simulink model "red4_16b"  (R2017a)
settings: Solver=VariableStepAuto  StartTime=0.0  StopTime=10.0  RelTol=1e-3
values from neighbouring files (symbols this model uses):
  alpha = 1    [red_parameters.m]
  beta = 0.7    [red_parameters.m]
  C_river = .017    (= 0.017)    [red_parameters.m]
  C_sea = 0.510    (= 0.51)    [red_parameters.m]
  F = 96485    [red_parameters.m]
  h_river = 60e-6    (= 6e-05)    [red_parameters.m]
  h_sea = 60e-6    (= 6e-05)    [red_parameters.m]
  k_river = 50e-3    (= 0.05)    [red_parameters.m]
  k_sea = 5    [red_parameters.m]
  L = 0.1    [red_parameters.m]
  m_v = 0.0008891    [red_parameters.m]
  Nm = 2    [red_parameters.m]
  R = 8.31    [red_parameters.m]
  R_AEM = R_cl    [red_parameters.m]
  R_CEM = R_Na    [red_parameters.m]
  R_electrodes = 2    [red_parameters.m]
  r_river = 1    [red_parameters.m]
  r_sea = 1    [red_parameters.m]
  SspVsp = 8/h_sea    (= 133333.333333)    [red_parameters.m]
  T = 298    [red_parameters.m]
  t_res = 100    [red_parameters.m]
  z = 1    [red_parameters.m]
undefined symbols (not defined in the file or in its folder): magnitude
libraries: fl_lib x6, nesl_utility x5
settings Model: Creator=root  LastModifiedBy=root

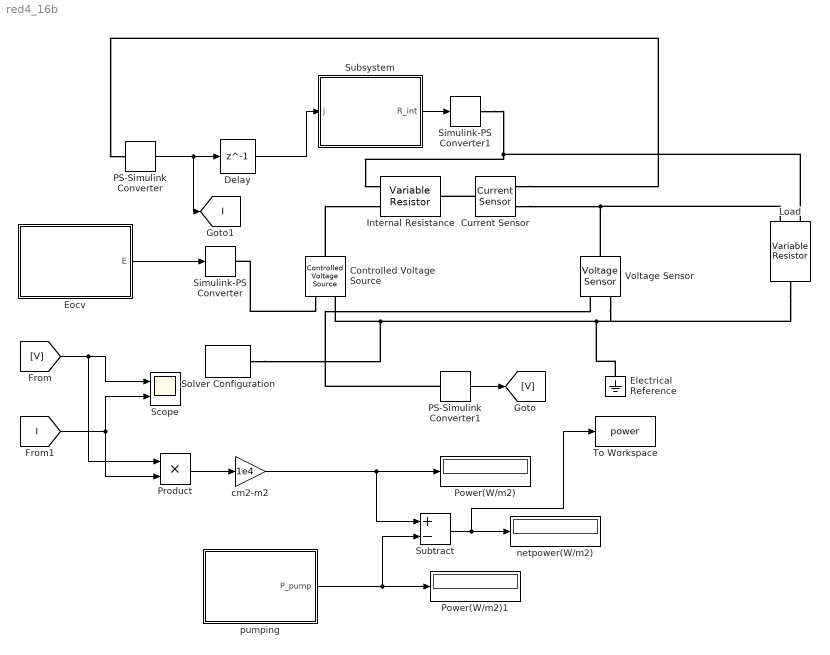
== system red4_16b ==
  Controlled Voltage Source : fl_lib/Electrical/Electrical Sources/Controlled Voltage Source
  Current Sensor : fl_lib/Electrical/Electrical Sensors/Current Sensor
  Delay : Delay  DelayLength=1  InitialCondition=0
  Electrical Reference : fl_lib/Electrical/Electrical Elements/Electrical Reference
  Eocv : Subsystem
  Internal Resistance : fl_lib/Electrical/Electrical Elements/Variable Resistor  Rmin=0 Ohm  i_specify=off  i_priority=None  i=0 A  i_nominal_specify=off  i_nominal_unit=A  i_nominal_value=1  v_specify=off  v_priority=None  v=0 V  v_nominal_specify=off  v_nominal_unit=V  v_nominal_value=1
  Load : fl_lib/Electrical/Electrical Elements/Variable Resistor  Rmin=0 Ohm  i_specify=off  i_priority=None  i=0 A  i_nominal_specify=off  i_nominal_unit=A  i_nominal_value=1  v_specify=off  v_priority=None  v=0 V  v_nominal_specify=off  v_nominal_unit=V  v_nominal_value=1
  PS-Simulink Converter : nesl_utility/PS-Simulink Converter  PhysicalDomain=network_engine_domain  SubClassName=ps_output  LeftPortType=input  RightPortType=output  PseudoPeriodic=off  Frequencies=[]  Unit=1  AffineConversion=off
  PS-Simulink Converter1 : nesl_utility/PS-Simulink Converter  PhysicalDomain=network_engine_domain  SubClassName=ps_output  LeftPortType=input  RightPortType=output  PseudoPeriodic=off  Frequencies=[]  Unit=1  AffineConversion=off
  Power(W/m2) : Display
  Power(W/m2)1 : Display
  Product : Product
  Scope : Scope  NumInputPorts=2
  Simulink-PS Converter : nesl_utility/Simulink-PS Converter  PhysicalDomain=network_engine_domain  SubClassName=ps_input  LeftPortType=input  RightPortType=output  PseudoPeriodic=off  Frequencies=[]  NoiseDistribution=none  NoiseParameters=[]  Unit=1  AffineConversion=off  FilteringAndDerivatives=provide  SimscapeFilterOrder=1  InputFilterTimeConstant=0.001  UdotUserProvided=0
  Simulink-PS Converter1 : nesl_utility/Simulink-PS Converter  PhysicalDomain=network_engine_domain  SubClassName=ps_input  LeftPortType=input  RightPortType=output  PseudoPeriodic=off  Frequencies=[]  NoiseDistribution=none  NoiseParameters=[]  Unit=1  AffineConversion=off  FilteringAndDerivatives=provide  SimscapeFilterOrder=1  InputFilterTimeConstant=0.001  UdotUserProvided=0
  Solver Configuration : nesl_utility/Solver Configuration  PhysicalDomain=network_engine_domain  SubClassName=solver  LeftPortType=input  RightPortType=generic  Accelerate=off  Tones=[]  Harmonics=[]  SimulateNoise=off  Profile=off  UseLocalSampling=off  EnableSwitchedLinearOptims=on  FrequencyDomain=off  UseCCode=off  RelTol=0.001  AbsTol=1e-06  MinStep=1e-09  ToWorkspace=off  RevertToSquareIcSolve=off  NumHomotopyIterations=100  PhasorMode=off  PhasorModeNumHarmonics=1  OverrideAbsTol=off  DoDC=off  ResidualTolerance=1e-09  UseLocalSolver=off  LocalSolverChoice=NE_BACKWARD_EULER_ADVANCER  LocalSolverSampleTime=0.001  DoFixedCost=off  MaxNonlinIter=3  MaxModeIter=2  LinearAlgebra=Sparse  DelaysMemoryBudget=1024  AutomaticFiltering=on  FilteringTimeConstant=0.001
  Subsystem : Subsystem
  Subtract : Sum  Inputs=+-
  To Workspace : ToWorkspace  VariableName=power  SampleTime=1
      settings: MaxDataPoints=1
  Voltage Sensor : fl_lib/Electrical/Electrical Sensors/Voltage Sensor
  cm2-m2 : Gain  Gain=1e4
  netpower(W/m2) : Display
  "pumping " : Subsystem
  tag scope: I=global
  wires:
  Eocv/1(E) -> Simulink-PS Converter/1
  Subsystem/1(R_int) -> Simulink-PS Converter1/1
  PS-Simulink Converter/1 -> [I], Delay/1
  Delay/1 -> Subsystem/1(j)
  PS-Simulink Converter1/1 -> [V]
  [V] -> Product/1, Scope/1
  [I] -> Product/2, Scope/2
  Product/1 -> cm2-m2/1
  cm2-m2/1 -> Subtract/1, Power(W/m2)/1
  "pumping "/1(P_pump) -> Subtract/2, Power(W/m2)1/1
  Subtract/1 -> To Workspace/1, netpower(W/m2)/1
  connections:
  Controlled Voltage Source/RConn1 -- Simulink-PS Converter/RConn1
  Simulink-PS Converter1/RConn1 -- Load/LConn1 -- Internal Resistance/LConn1
  Controlled Voltage Source/LConn1 -- Internal Resistance/LConn2
  Load/RConn1 -- Voltage Sensor/RConn2 -- Electrical Reference/LConn1 -- Solver Configuration/RConn1 -- Controlled Voltage Source/RConn2
  Current Sensor/LConn1 -- Internal Resistance/RConn1
  Current Sensor/RConn2 -- Load/LConn2 -- Voltage Sensor/LConn1
  Current Sensor/RConn1 -- PS-Simulink Converter/LConn1
  PS-Simulink Converter1/LConn1 -- Voltage Sensor/RConn1

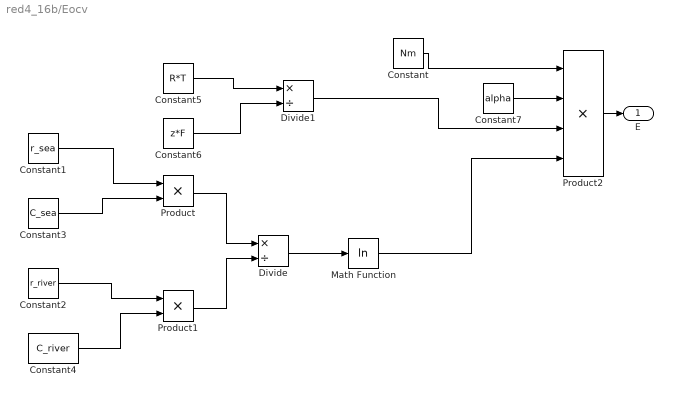
== system red4_16b/Eocv ==
  Constant : Constant  Value=Nm
  Constant1 : Constant  Value=r_sea
  Constant2 : Constant  Value=r_river
  Constant3 : Constant  Value=C_sea
  Constant4 : Constant  Value=C_river
  Constant5 : Constant  Value=R*T
  Constant6 : Constant  Value=z*F
  Constant7 : Constant  Value=alpha
  Divide : Product  Inputs=*/
  Divide1 : Product  Inputs=*/
  Math Function : Math  Operator=log  SaturateOnIntegerOverflow=on
  Product : Product
  Product1 : Product
  Product2 : Product  Inputs=4
  E : Outport
  wires:
  Constant5/1 -> Divide1/1
  Constant1/1 -> Product/1
  Constant4/1 -> Product1/2
  Constant3/1 -> Product/2
  Constant2/1 -> Product1/1
  Product/1 -> Divide/1
  Divide/1 -> Math Function/1
  Product1/1 -> Divide/2
  Constant6/1 -> Divide1/2
  Divide1/1 -> Product2/3
  Math Function/1 -> Product2/4
  Product2/1 -> E/1
  Constant/1 -> Product2/1
  Constant7/1 -> Product2/2

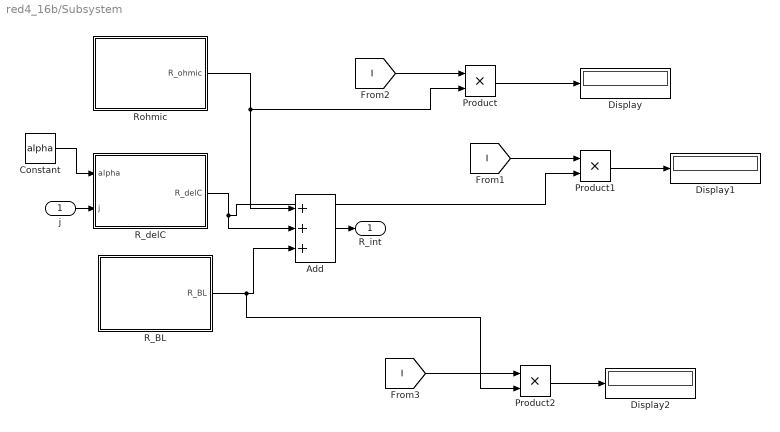
== system red4_16b/Subsystem ==
  j : Inport
  Add : Sum  Inputs=3
  Constant : Constant  Value=alpha
  Display : Display
  Display1 : Display
  Display2 : Display
  Product : Product
  Product1 : Product
  Product2 : Product
  R_BL : Subsystem
  R_delC : Subsystem
  Rohmic : Subsystem
  R_int : Outport
  wires:
  Constant/1 -> R_delC/1(alpha)
  Rohmic/1(R_ohmic) -> Product/2, Add/1
  j/1 -> R_delC/2(j)
  Add/1 -> R_int/1
  [I] -> Product/1
  [I] -> Product1/1
  R_delC/1(R_delC) -> Product1/2, Add/2
  [I] -> Product2/1
  R_BL/1(R_BL) -> Product2/2, Add/3
  Product/1 -> Display/1
  Product1/1 -> Display1/1
  Product2/1 -> Display2/1

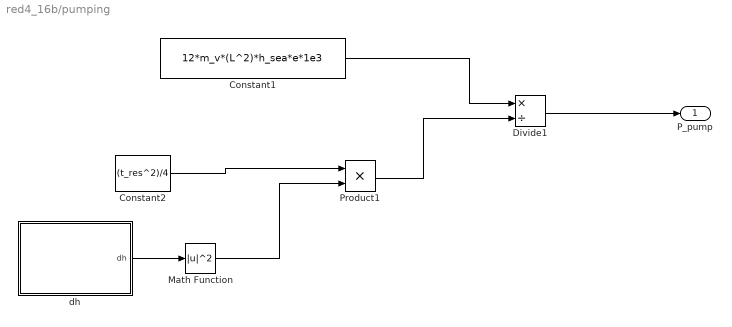
== system red4_16b/pumping  ==
  Constant1 : Constant  Value=12*m_v*(L^2)*h_sea*e*1e3
  Constant2 : Constant  Value=(t_res^2)/4
  Divide1 : Product  Inputs=*/
  Math Function : Math  Operator=magnitude^2  SaturateOnIntegerOverflow=on
  Product1 : Product
  dh : Subsystem
  P_pump : Outport
  wires:
  Constant1/1 -> Divide1/1
  Constant2/1 -> Product1/1
  Product1/1 -> Divide1/2
  dh/1(dh) -> Math Function/1
  Math Function/1 -> Product1/2
  Divide1/1 -> P_pump/1

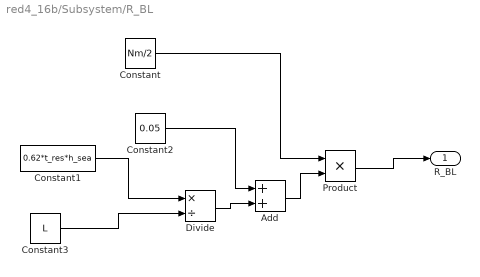
== system red4_16b/Subsystem/R_BL ==
  Add : Sum
  Constant : Constant  Value=Nm/2
  Constant1 : Constant  Value=0.62*t_res*h_sea
  Constant2 : Constant  Value=0.05
  Constant3 : Constant  Value=L
  Divide : Product  Inputs=*/
  Product : Product
  R_BL : Outport
  wires:
  Constant1/1 -> Divide/1
  Constant3/1 -> Divide/2
  Divide/1 -> Add/2
  Constant2/1 -> Add/1
  Add/1 -> Product/2
  Constant/1 -> Product/1
  Product/1 -> R_BL/1

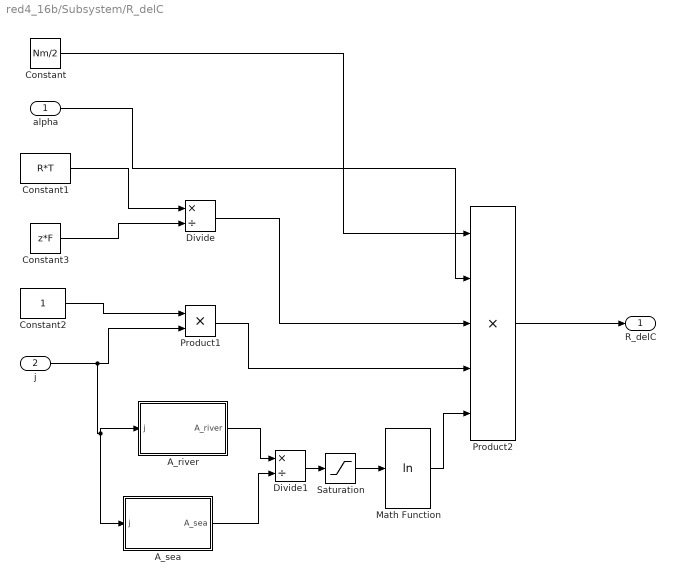
== system red4_16b/Subsystem/R_delC ==
  alpha : Inport
  j : Inport  Port=2
  A_river : Subsystem
  A_sea : Subsystem
  Constant : Constant  Value=Nm/2
  Constant1 : Constant  Value=R*T
  Constant2 : Constant
  Constant3 : Constant  Value=z*F
  Divide : Product  Inputs=*/
  Divide1 : Product  Inputs=*/
  Math Function : Math  Operator=log  SaturateOnIntegerOverflow=on
  Product1 : Product
  Product2 : Product  Inputs=5
  Saturation : Saturate  UpperLimit=inf  LowerLimit=0.001
  R_delC : Outport
  wires:
  Constant1/1 -> Divide/1
  j/1 -> A_sea/1(j), A_river/1(j), Product1/2
  Constant3/1 -> Divide/2
  Constant2/1 -> Product1/1
  A_river/1(A_river) -> Divide1/1
  A_sea/1(A_sea) -> Divide1/2
  Divide1/1 -> Saturation/1
  Constant/1 -> Product2/1
  alpha/1 -> Product2/2
  Divide/1 -> Product2/3
  Product1/1 -> Product2/4
  Math Function/1 -> Product2/5
  Product2/1 -> R_delC/1
  Saturation/1 -> Math Function/1

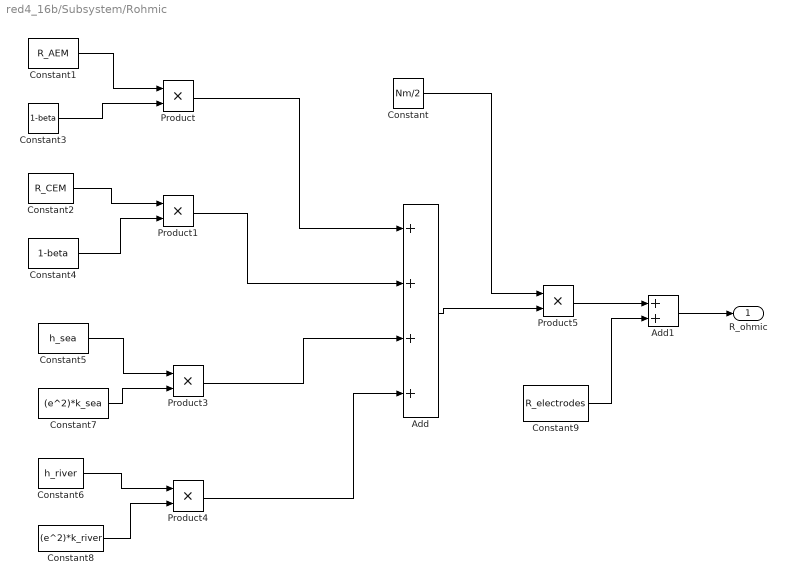
== system red4_16b/Subsystem/Rohmic ==
  Add : Sum  Inputs=4
  Add1 : Sum
  Constant : Constant  Value=Nm/2
  Constant1 : Constant  Value=R_AEM
  Constant2 : Constant  Value=R_CEM
  Constant3 : Constant  Value=1-beta
  Constant4 : Constant  Value=1-beta
  Constant5 : Constant  Value=h_sea
  Constant6 : Constant  Value=h_river
  Constant7 : Constant  Value=(e^2)*k_sea
  Constant8 : Constant  Value=(e^2)*k_river
  Constant9 : Constant  Value=R_electrodes
  Product{,1,3..5} (5 alike) : Product
  R_ohmic : Outport
  wires:
  Constant1/1 -> Product/1
  Constant4/1 -> Product1/2
  Constant3/1 -> Product/2
  Constant2/1 -> Product1/1
  Add1/1 -> R_ohmic/1
  Constant5/1 -> Product3/1
  Constant6/1 -> Product4/1
  Constant7/1 -> Product3/2
  Constant8/1 -> Product4/2
  Product/1 -> Add/1
  Product1/1 -> Add/2
  Product3/1 -> Add/3
  Product4/1 -> Add/4
  Constant/1 -> Product5/1
  Add/1 -> Product5/2
  Product5/1 -> Add1/1
  Constant9/1 -> Add1/2

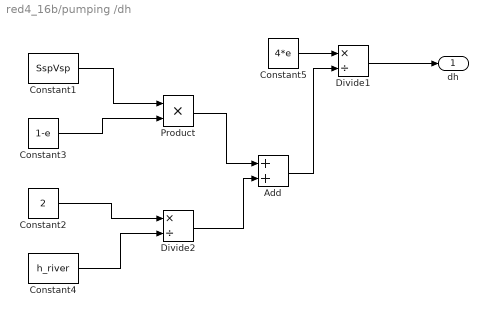
== system red4_16b/pumping /dh ==
  Add : Sum
  Constant1 : Constant  Value=SspVsp
  Constant2 : Constant  Value=2
  Constant3 : Constant  Value=1-e
  Constant4 : Constant  Value=h_river
  Constant5 : Constant  Value=4*e
  Divide1 : Product  Inputs=*/
  Divide2 : Product  Inputs=*/
  Product : Product
  dh : Outport
  wires:
  Constant5/1 -> Divide1/1
  Constant1/1 -> Product/1
  Constant4/1 -> Divide2/2
  Constant3/1 -> Product/2
  Constant2/1 -> Divide2/1
  Product/1 -> Add/1
  Divide2/1 -> Add/2
  Add/1 -> Divide1/2
  Divide1/1 -> dh/1

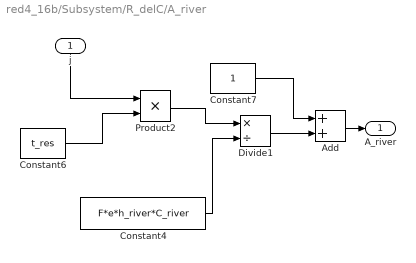
== system red4_16b/Subsystem/R_delC/A_river ==
  j : Inport
  Add : Sum
  Constant4 : Constant  Value=F*e*h_river*C_river
  Constant6 : Constant  Value=t_res
  Constant7 : Constant
  Divide1 : Product  Inputs=*/
  Product2 : Product
  A_river : Outport
  wires:
  Constant7/1 -> Add/1
  Product2/1 -> Divide1/1
  Constant4/1 -> Divide1/2
  Add/1 -> A_river/1
  Constant6/1 -> Product2/2
  j/1 -> Product2/1
  Divide1/1 -> Add/2

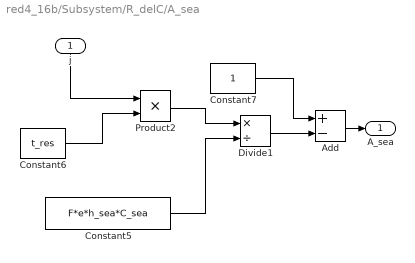
== system red4_16b/Subsystem/R_delC/A_sea ==
  j : Inport
  Add : Sum  Inputs=+-
  Constant5 : Constant  Value=F*e*h_sea*C_sea
  Constant6 : Constant  Value=t_res
  Constant7 : Constant
  Divide1 : Product  Inputs=*/
  Product2 : Product
  A_sea : Outport
  wires:
  Constant7/1 -> Add/1
  Product2/1 -> Divide1/1
  Constant5/1 -> Divide1/2
  Add/1 -> A_sea/1
  Constant6/1 -> Product2/2
  j/1 -> Product2/1
  Divide1/1 -> Add/2
